simulink model "2ndOrderSingleBitSC"  (R2012b)
settings: Solver=VariableStepDiscrete  StartTime=0.0  StopTime=(N-1)*ts  RelTol=1e-3
values from neighbouring files (symbols this model uses):
  Adc = 10.^(1+2*rand(1,n_sim))    [sim211CascadeSDM.m]    (also in sim2ndSCSDM.m; sim2ndSCmultibitSDM.m)
  Ain = 0.5    [211CascadeSDM.mat]    (also in GeneralParams211CascadeSDM.m; GeneralParams2orSCSDM.m; GeneralParams2orSCmultibitSDM.m)
  cs1a = 10e-12    (= 1e-11)    [GeneralParams2orSCSDM.m]    (also in GeneralParams2orSCmultibitSDM.m)
  f = rand(3,1)*0.8+0.2    [sim211CascadeSDM.m]
  fin = Bw./5    [sim2ndSCSDM.m]    (also in sim2ndSCmultibitSDM.m)
  gm = 10.^(-5+2*rand(1,n_sim))    [sim211CascadeSDM.m]    (also in sim2ndSCSDM.m; sim2ndSCmultibitSDM.m)
  io = 10.^(-4+2*rand(1,n_sim))    [sim211CascadeSDM.m]    (also in sim2ndSCSDM.m; sim2ndSCmultibitSDM.m)
  N = 65536    [211CascadeSDM.mat]    (also in GeneralParams211CascadeSDM.m; GeneralParams2orSCSDM.m; GeneralParams2orSCmultibitSDM.m)
  ts = 1./fs    [sim211CascadeSDM.m]    (also in sim2ndSCSDM.m; sim2ndSCmultibitSDM.m; sim3or21CascadeSCSDM.m)
  Vn = 10.^(-11+4*rand(1,n_sim))    [sim2ndSCSDM.m]    (also in sim2ndSCmultibitSDM.m)
  vosp = 5    [211CascadeSDM.mat]    (also in GeneralParams211CascadeSDM.m; GeneralParams2orSCSDM.m; GeneralParams2orSCmultibitSDM.m)
undefined symbols (not defined in the file or in its folder): FH, FL, sinker
undefined symbols (not defined in the file): fs, M
libraries: fesclib x2, quantidlib x1
settings Model: SimulationMode=accelerator  Creator=jrosa  LastModifiedBy=Beatriz
settings OptimizationCC: InlineInvariantSignals=on  InitFltsAndDblsToZero=on
settings DebuggingCC: SaveWithParameterizedLinksMsg=none  SignalResolutionControl=TryResolveAllWithWarning  MultiTaskDSMMsg=warning  MultiTaskCondExecSysMsg=none  FcnCallInpInsideContextMsg=UseLocalSettings  StrictBusMsg=None
settings RTWCC: IncludeERTFirstTime=on
settings GRTTargetCC: TargetFcnLib=ansi_tfl_tmw.mat  CombineOutputUpdateFcns=off  GRTInterface=on

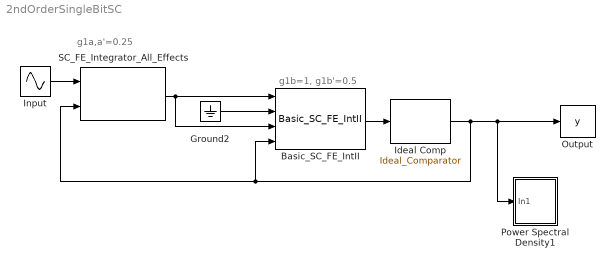
== system 2ndOrderSingleBitSC ==
  note: g1a,a'=0.25
  note: g1b=1, g1b'=0.5
  Basic_SC_FE_IntII : fesclib/Basic_SC_FE_IntII  opspos=vosp  opsneg=-vosp  c2=ci1b  c11=cs1b  c12=cs1b  phi=phi1  ts=ts
  Ground2 : Ground
  Ideal Comp : quantidlib/Ideal_Comparator  Vhigh=vhigh  Vlow=vlow  phi=phi1  ts=ts  qid=cuant1G
      link override Goto: GotoTag=cuant1G
  Input : Sin  Amplitude=Ain  Frequency=2*pi*fin  SampleTime=0
  Output : ToWorkspace  VariableName=y  SampleTime=ts
  Power Spectral Density1 : Subsystem  AncestorBlock=SDtoolbox/Power Spectral Density  mask{SN=2, Fs=fs, fBL=1, fBH=fs/M, Fin=fin, N=N, Ntransient=0, VW=off, savename=savemat, Scale_type=linear}
      mask prompts: SN "Scope Number"; Fs "Sampling Frequency [Hz]"; fBL "Lower Band Bound [Hz]"; fBH "Upper Band Bound [Hz]"; Fin "Signal Frequency [Hz]"; N "Number of FFT Points"; Ntransient "Number of Transient Points"; VW "Variables Available in the Workspace"; savename "Nome of .mat File"; Scale_type "Scale"
      mask help: Calculates power spectral density, signal-to-noise ratio and effective number of bits of the Sigma-Delta modulator output
      mask init:
      | [f,FL,FH]=sinker_ini(Fs,fBL,fBH,Fin,N,SN);
      mask Help: web('PSD.html','-helpbrowser')
      mask Callback VW:
      | opt1=(get_param(gcb,'VW'));
      | switch opt1
      | 	case 'off'
      | 				set_param(gcb,'MaskEnables',{'on','on','on','on','on','on','on','on','off','on'});
      | 	case 'on'
      | 				set_param(gcb,'MaskEnables',{'on','on','on','on','on','on','on','on','on','on'});
      | end
      mask TypeOptions Scale_type: linear | logarithmic
      mask Display:
      | plot(0,0,1,1,[.14,.91,.91,.14,.14],[.86,.86,.40,.40,.86],[.85,.82,.80,.79,.75,.67,.63,.60,.57,.53,.41,.36,.33,.27,.24],[.49,.50,.53,.50,.49,.51,.54,.63,.54,.50,.50,.52,.82,.52,.45])
      | text(.54,.18, 'PSD','horizontalAlignment', 'center')
  SC_FE_Integrator_All_Effects : fesclib/SC_FE_Integrator_All_Effects  c=[cs1a,4*cs1a,0,0]  var=[0,Vn,275,300]  ops=[vosp,-vosp]  ao=[Adc,gm,io]  avnl=[0,0,0,0]  cp=[0.05e-12,0.05e-12,2.5e-12]  phi=phi1  ts=ts  settlingon=on  setin=off  idown=int1  idnext=int1
      link override Capacidades: Value=1e-11
      link override From: GotoTag=int1
      link override Goto: GotoTag=int1
  wires:
  Basic_SC_FE_IntII/1 -> Ideal Comp/1
  Ground2/1 -> Basic_SC_FE_IntII/2
  SC_FE_Integrator_All_Effects/1 -> Basic_SC_FE_IntII/1, Basic_SC_FE_IntII/3
  Input/1 -> SC_FE_Integrator_All_Effects/1
  Ideal Comp/1 -> Basic_SC_FE_IntII/4, SC_FE_Integrator_All_Effects/2, Power Spectral Density1/1(In1), Output/1

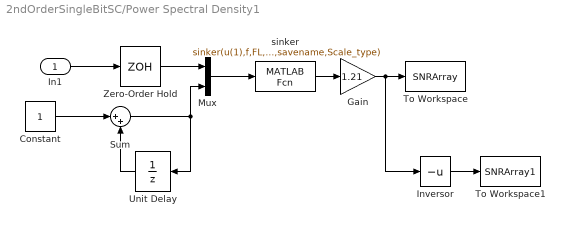
== system 2ndOrderSingleBitSC/Power Spectral Density1 ==
  In1 : Inport
  Constant : Constant
  Gain : Gain  Gain=1.21
  Inversor : UnaryMinus
  Mux : Mux  Inputs=2
  Sum : Sum  Inputs=|++  SaturateOnIntegerOverflow=on
  To Workspace : ToWorkspace  VariableName=SNRArray  SampleTime=-1
      settings: MaxDataPoints=1
  To Workspace1 : ToWorkspace  VariableName=SNRArray1  SampleTime=-1
      settings: MaxDataPoints=1
  Unit Delay : UnitDelay  SampleTime=1/Fs
  Zero-Order Hold : ZeroOrderHold  SampleTime=1/Fs
  sinker : MATLABFcn  MATLABFcn=sinker(u(1),f,FL,FH,N,Ntransient,u(2),SN,Fs,VW,savename,Scale_type)
  wires:
  Zero-Order Hold/1 -> Mux/1
  In1/1 -> Zero-Order Hold/1
  Mux/1 -> sinker/1
  Sum/1 -> Mux/2, Unit Delay/1
  Constant/1 -> Sum/1
  Unit Delay/1 -> Sum/2
  sinker/1 -> Gain/1
  Inversor/1 -> To Workspace1/1
  Gain/1 -> To Workspace/1, Inversor/1
